simulink model "Sistema_no_Lineal_Validacion"  (R2016a)
settings: Solver=VariableStepAuto  StartTime=0.0  StopTime=10.0  RelTol=1e-3
undefined symbols (not defined in the file or in its folder): Theta
settings Model: Creator=Daniel  LastModifiedBy=Daniel

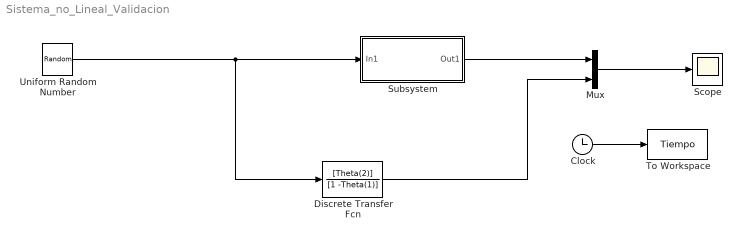
== system Sistema_no_Lineal_Validacion ==
  Clock : Clock
  Discrete Transfer Fcn : DiscreteTransferFcn  Numerator=[Theta(2)]  Denominator=[1 -Theta(1)]  SampleTime=0.01
  Mux : Mux  Inputs=2
  Scope : Scope
  Subsystem : Subsystem
  To Workspace : ToWorkspace  VariableName=Tiempo  SampleTime=0.01
  Uniform Random Number : UniformRandomNumber  Minimum=0  Maximum=5  SampleTime=0.05
  wires:
  Uniform Random Number/1 -> Discrete Transfer Fcn/1, Subsystem/1(In1)
  Subsystem/1(Out1) -> Mux/1
  Mux/1 -> Scope/1
  Clock/1 -> To Workspace/1
  Discrete Transfer Fcn/1 -> Mux/2

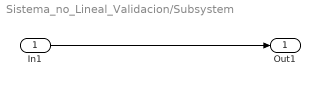
== system Sistema_no_Lineal_Validacion/Subsystem ==
  In1 : Inport  SampleTime=0.01
  Out1 : Outport  SampleTime=0.01
  wires:
  In1/1 -> Out1/1
